simulink library "ilcUpdateLaw_cl"  (R2018b)
settings: Solver=VariableStepAuto  StartTime=0.0  StopTime=10.0  RelTol=1e-3
libraries: simulink x1
settings Model: Creator=mcobb  LastModifiedBy=mcobb

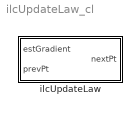
== system ilcUpdateLaw_cl ==
  ilcUpdateLaw : Subsystem  mask{lrn=0, trstRgn=0, wtNoise=0}
      mask prompts: lrn "Gradient Based Learning Gain"; trstRgn "Trust Region Dimensions"; wtNoise "White Noise Dimensions"

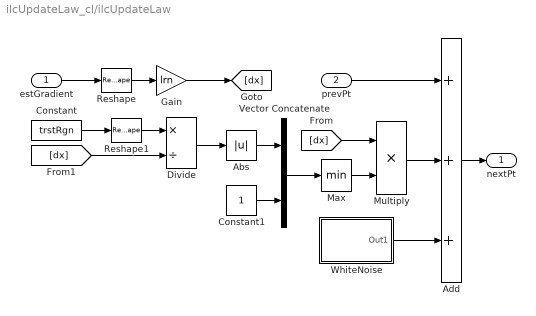
== system ilcUpdateLaw_cl/ilcUpdateLaw ==
  estGradient : Inport
  prevPt : Inport  Port=2
  Abs : Abs
  Add : Sum  Inputs=+++
  Constant : Constant  Value=trstRgn
  Constant1 : Constant
  Divide : Product  Inputs=*/
  Gain : Gain  Gain=lrn
  Max : MinMax
  Multiply : Product
  Reshape : Reshape  OutputDimensionality=Column vector (2-D)
  Reshape1 : Reshape  OutputDimensionality=Column vector (2-D)
  Vector Concatenate : Concatenate
  WhiteNoise : Subsystem  TreatAsAtomicUnit=on  mask{seeds=0, amps=0}
      mask prompts: seeds "Noise Seeds"; amps "Noise Amplitudes"
  nextPt : Outport
  wires:
  prevPt/1 -> Add/1
  estGradient/1 -> Reshape/1
  Multiply/1 -> Add/2
  [dx] -> Multiply/1
  Reshape/1 -> Gain/1
  Divide/1 -> Abs/1
  [dx] -> Divide/2
  Constant/1 -> Reshape1/1
  Reshape1/1 -> Divide/1
  WhiteNoise/1(Out1) -> Add/3
  Add/1 -> nextPt/1
  Gain/1 -> [dx]
  Max/1 -> Multiply/2
  Constant1/1 -> Vector Concatenate/2
  Vector Concatenate/1 -> Max/1
  Abs/1 -> Vector Concatenate/1

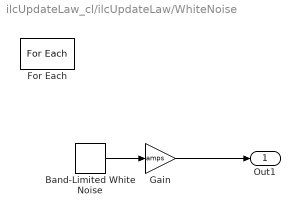
== system ilcUpdateLaw_cl/ilcUpdateLaw/WhiteNoise ==
  Band-Limited White Noise : simulink/Sources/Band-Limited White Noise  Cov=[0.1]  Ts=1  seed=seeds
  For Each : ForEach  DisableCoverage=on  IterateSubsysMaskParameter=on,on  SubsysMaskParameterIterationDimension=2,2  IndexMode=One-based
  Gain : Gain  Gain=amps
  Out1 : Outport  ConcatenationDimension=1
  wires:
  Band-Limited White Noise/1 -> Gain/1
  Gain/1 -> Out1/1
